simulink library "MuteRamperBtc"  (R2022b)
settings: Solver=VariableStepAuto  StartTime=0.0  StopTime=10.0  RelTol=1e-3
undefined symbols (not defined in the file or in its folder): InnerLinkConfig
libraries: AudioStats x1, FeaturePath x1, HandyTextFile x1, dspindex x1
settings Model: Creator=kl13806  LastModifiedBy=db1045444
settings SolverCC: AlgebraicLoopSolver=TrustRegion
settings DebuggingCC: UnconnectedInputMsg=warning  UnconnectedOutputMsg=warning  UnconnectedLineMsg=warning  SFMachineParentedDataDiag=warning
settings ModelReferenceCC: EnableRefExpFcnMdlSchedulingChecks=on
settings RTWCC: DLArmComputeVersion=19.05

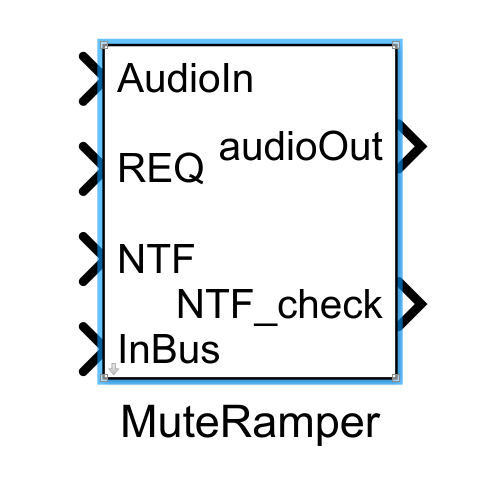
[thumbnail: Simulink's stored preview of the top-level diagram]
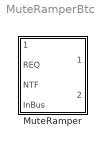
== system MuteRamperBtc ==
  MuteRamper : Subsystem  mask(Blocklib MuteRamper){Config=InnerLinkConfig, FeatureName=Mute}
      mask prompts: Config "MuteRamperConfig"; FeatureName "Feature path name:"
      mask help: This component is to be used in conjunction with the MuteControl block, which provides runtime control and tuning capabilities via an RTC and the tune variable muteControlRampTime. Multiple instances of this block may be placed within an audio application, and a single MuteControl block has the ability to control all of these rampers simultaneously.
      mask init:
      | blkh=gcbh;
      | Config=BTConfig.Assert(blkh,Config);
      | Config.Validate();
      | 
      | % Set boundary conditions
      | rampRateBounds = [5,50000];
      | rampTimeBounds = [1,3000];
      | 
      | % Setup Dsms
      | theDsms = {'currentGain','targetLinearGain','nFrames'};
      | CscUtil.SetupDsmsForStaticInit(blkh,theDsms);
      mask TypeOptions FeatureName: FeaturePath/FeatureName

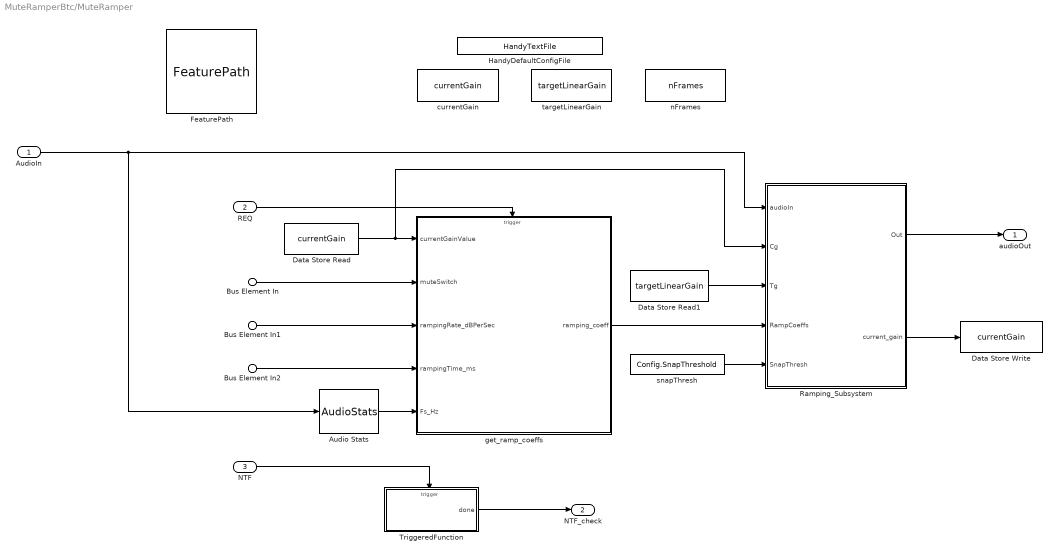
== system MuteRamperBtc/MuteRamper ==
  AudioIn : Inport
  REQ : Inport  Port=2
  NTF : Inport  Port=3
  Bus Element In : Inport  Port=4  PortName=InBus  Element=REQ_mute_switch
  Bus Element In1 : Inport  Port=4  PortName=InBus  Element=rampRate
  Bus Element In2 : Inport  Port=4  PortName=InBus  Element=rampTime
  Audio Stats : AudioStats/AudioStats  DoSampleRate=on  TypeSampleRate=Inherit: auto  DoCallRate=off  TypeCallRate=Inherit: auto  DoFrameSize=off  TypeFrameSize=Inherit: auto  DoChannelCount=off  TypeChannelCount=Inherit: auto  DoTaskRateFactor=off  TypeTaskRateFactor=Inherit: auto  MacroNameRoot=AUDIO  MacroNameRootEval='AUDIO'  IsMacroNameEval=off  MacroSampleRate=off  MacroCallRate=off  MacroFrameSize=off  MacroChannelCount=off  MacroTaskRateFactor=off  MacroTaskId=off  ValidateSampleRate=off  ValueSampleRate=[]  ValidateCallRate=off  ValueCallRate=[]  ValidateFrameSize=off  ValueFrameSize=[]  ValidateChannelCount=off  ValueChannelCount=[]  ValidateTaskRateFactor=off  ValueTaskRateFactor=[]
      settings: SourceProductName=Bose Talaria
  Data Store Read : DataStoreRead  DataStoreName=currentGain  IndexOptions=Index vector (dialog)  Indices=1  OutputSizes=1
  Data Store Read1 : DataStoreRead  DataStoreName=targetLinearGain  IndexOptions=Index vector (dialog)  Indices=1  OutputSizes=1
  Data Store Write : DataStoreWrite  DataStoreName=currentGain  IndexOptions=Index vector (dialog)  Indices=1  OutputSizes=1
  FeaturePath : FeaturePath/FeaturePath  FeatureName=Mute  IsGroup=off  GroupNumber=-1  IsModule=off  TriggerInit=[640 -31 755 76]
      settings: SourceProductName=Bose Talaria
  HandyDefaultConfigFile : HandyTextFile/HandyTextFile  TemplateSource=Config  FileSuffix=Init  OpenDialogOnLoad=off  UseThisBlockName=off  AddGrandParentNamePrefix=off  TheDefaultText=|  ShowInLibBrowser=on
      | % $(FILENAME) Setup model parameters for each "Init" callback (e.g. update diagram)
      | sample_rate_in_hertz = 44100;
      | frame_size = 32;
      | sysin_channel_count = 2;
      settings: SourceProductName=Bose Talaria
  Ramping_Subsystem : Subsystem  TreatAsAtomicUnit=on
  TriggeredFunction : MATLAB Function  TreatAsAtomicUnit=on
  currentGain : DataStoreMemory  DataStoreName=currentGain  InitialValue=Config.DlgInitialGainLinear  ShowAdditionalParam=off  OutDataTypeStr=single
  get_ramp_coeffs : MATLAB Function  TreatAsAtomicUnit=on  mask{silentGainLinear=Config.SilentGainLinear, frameSize=Config.SamplesPerFrame}
  nFrames : DataStoreMemory  DataStoreName=nFrames  ShowAdditionalParam=off  OutDataTypeStr=single
  snapThresh : Constant  Value=Config.SnapThreshold  VectorParams1D=off  OutDataTypeStr=single
  targetLinearGain : DataStoreMemory  DataStoreName=targetLinearGain  InitialValue=Config.DlgInitialGainLinear  ShowAdditionalParam=off  OutDataTypeStr=single
  audioOut : Outport  VectorParamsAs1DForOutWhenUnconnected=off
  NTF_check : Outport  Port=2
  wires:
  REQ/1 -> get_ramp_coeffs/Trigger
  snapThresh/1 -> Ramping_Subsystem/5(SnapThresh)
  Audio Stats/1 -> get_ramp_coeffs/5(Fs_Hz)
  NTF/1 -> TriggeredFunction/Trigger
  TriggeredFunction/1(done) -> NTF_check/1
  Bus Element In/1 -> get_ramp_coeffs/2(muteSwitch)
  Ramping_Subsystem/2(current_gain) -> Data Store Write/1
  Bus Element In2/1 -> get_ramp_coeffs/4(rampingTime_ms)
  Data Store Read1/1 -> Ramping_Subsystem/3(Tg)
  get_ramp_coeffs/1(ramping_coeff) -> Ramping_Subsystem/4(RampCoeffs)
  Ramping_Subsystem/1(Out) -> audioOut/1
  AudioIn/1 -> Audio Stats/1, Ramping_Subsystem/1(audioIn)
  Bus Element In1/1 -> get_ramp_coeffs/3(rampingRate_dBPerSec)
  Data Store Read/1 -> Ramping_Subsystem/2(Cg), get_ramp_coeffs/1(currentGainValue)

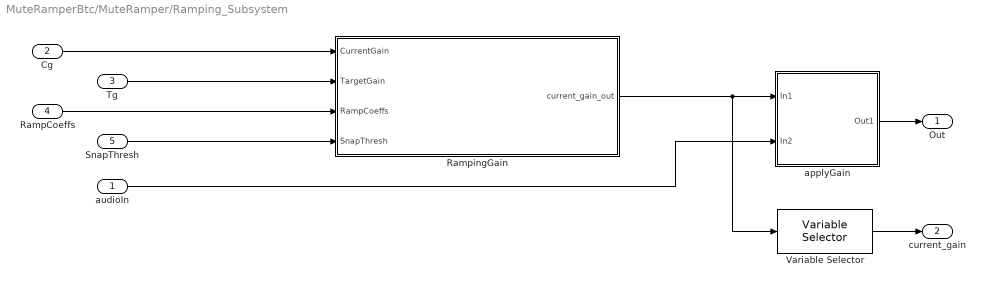
== system MuteRamperBtc/MuteRamper/Ramping_Subsystem ==
  audioIn : Inport
  Cg : Inport  Port=2
  Tg : Inport  Port=3
  RampCoeffs : Inport  Port=4
  SnapThresh : Inport  Port=5
  RampingGain : Subsystem
  Variable Selector : dspindex/Variable Selector  NumInputs=1  rowsOrCols=Rows  IdxMode=Fixed  Elements=Config.SamplesPerFrame  ZerOneIdxMode=One-based  errmode=Clip Index  FillMode=on  FillValues=0
  applyGain : Subsystem
  Out : Outport  VectorParamsAs1DForOutWhenUnconnected=off
  current_gain : Outport  Port=2  VectorParamsAs1DForOutWhenUnconnected=off
  wires:
  RampingGain/1(current_gain_out) -> applyGain/1(In1), Variable Selector/1
  audioIn/1 -> applyGain/2(In2)
  applyGain/1(Out1) -> Out/1
  Variable Selector/1 -> current_gain/1
  Cg/1 -> RampingGain/1(CurrentGain)
  SnapThresh/1 -> RampingGain/4(SnapThresh)
  Tg/1 -> RampingGain/2(TargetGain)
  RampCoeffs/1 -> RampingGain/3(RampCoeffs)

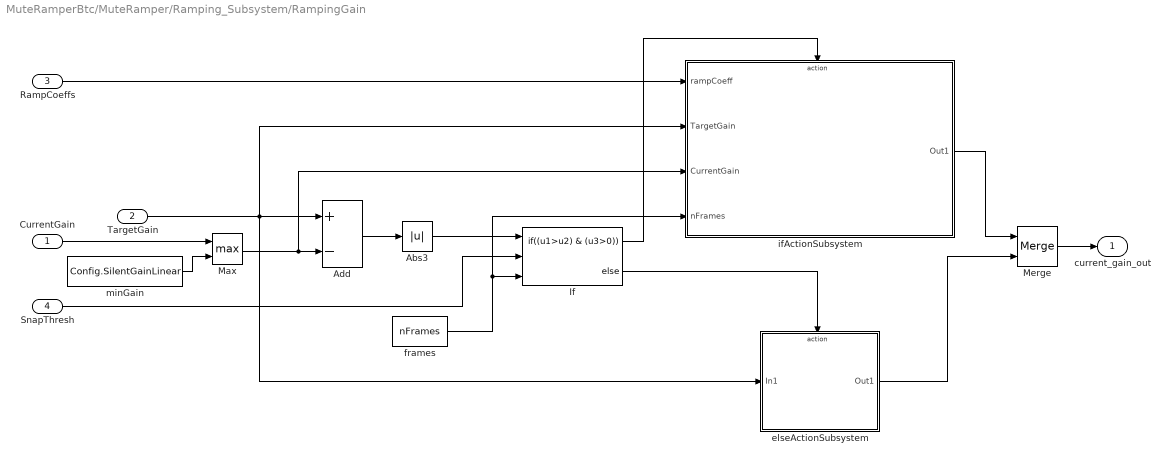
== system MuteRamperBtc/MuteRamper/Ramping_Subsystem/RampingGain ==
  CurrentGain : Inport
  TargetGain : Inport  Port=2
  RampCoeffs : Inport  Port=3
  SnapThresh : Inport  Port=4
  Abs3 : Abs  SaturateOnIntegerOverflow=off
  Add : Sum  Inputs=+-
  If : If  NumInputs=3  IfExpression=(u1>u2) & (u3>0)
  Max : MinMax  Function=max  Inputs=2
  Merge : Merge
  elseActionSubsystem : Subsystem
  frames : DataStoreRead  DataStoreName=nFrames  IndexOptions=Index vector (dialog)  Indices=1  OutputSizes=1
  ifActionSubsystem : Subsystem
  minGain : Constant  Value=Config.SilentGainLinear  OutDataTypeStr=single
  current_gain_out : Outport  VectorParamsAs1DForOutWhenUnconnected=off
  wires:
  Max/1 -> ifActionSubsystem/3(CurrentGain), Add/2
  Merge/1 -> current_gain_out/1
  Add/1 -> Abs3/1
  TargetGain/1 -> ifActionSubsystem/2(TargetGain), Add/1, elseActionSubsystem/1(In1)
  SnapThresh/1 -> If/2
  Abs3/1 -> If/1
  minGain/1 -> Max/2
  CurrentGain/1 -> Max/1
  If/1 -> ifActionSubsystem/Action
  If/2 -> elseActionSubsystem/Action
  RampCoeffs/1 -> ifActionSubsystem/1(rampCoeff)
  ifActionSubsystem/1(Out1) -> Merge/1
  elseActionSubsystem/1(Out1) -> Merge/2
  frames/1 -> ifActionSubsystem/4(nFrames), If/3

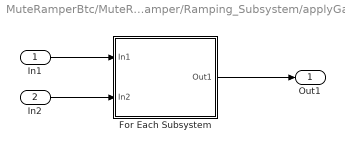
== system MuteRamperBtc/MuteRamper/Ramping_Subsystem/applyGain ==
  In1 : Inport
  In2 : Inport  Port=2
  For Each Subsystem : Subsystem  TreatAsAtomicUnit=on
  Out1 : Outport  VectorParamsAs1DForOutWhenUnconnected=off
  wires:
  In2/1 -> For Each Subsystem/2(In2)
  For Each Subsystem/1(Out1) -> Out1/1
  In1/1 -> For Each Subsystem/1(In1)

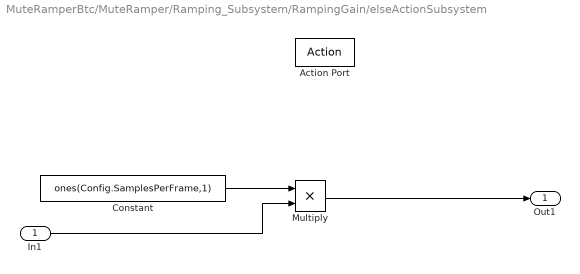
== system MuteRamperBtc/MuteRamper/Ramping_Subsystem/RampingGain/elseActionSubsystem ==
  In1 : Inport
  Action Port : ActionPort
  Constant : Constant  Value=ones(Config.SamplesPerFrame,1)  VectorParams1D=off  OutDataTypeStr=single
  Multiply : Product
  Out1 : Outport  VectorParamsAs1DForOutWhenUnconnected=off
  wires:
  Multiply/1 -> Out1/1
  In1/1 -> Multiply/2
  Constant/1 -> Multiply/1

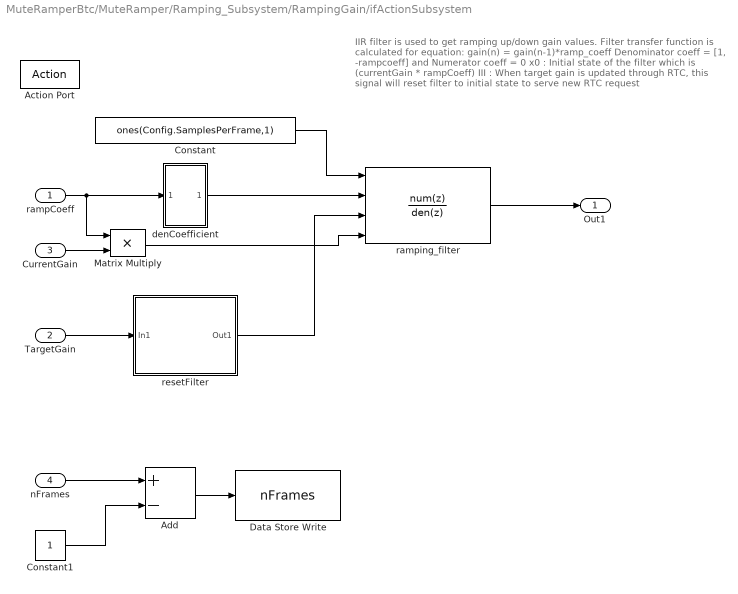
== system MuteRamperBtc/MuteRamper/Ramping_Subsystem/RampingGain/ifActionSubsystem ==
  note: IIR filter is used to get ramping up/down gain values. Filter transfer function
      |  is calculated for equation:
      | 	gain(n) = gain(n-1)*ramp_coeff
      |
      | Denominator coeff  = [1, -rampcoeff]  and Numerator coeff = 0
      | x0 : Initial state of the filter which is (currentGain * rampCoeff)
      | III : When target gain is updated through RTC, this signal will reset filter to
      | 	initial state to serve new RTC request
  rampCoeff : Inport
  TargetGain : Inport  Port=2
  CurrentGain : Inport  Port=3
  nFrames : Inport  Port=4
  Action Port : ActionPort
  Add : Sum  Inputs=+-
  Constant : Constant  Value=ones(Config.SamplesPerFrame,1)  VectorParams1D=off  OutDataTypeStr=single
  Constant1 : Constant  OutDataTypeStr=single
  Data Store Write : DataStoreWrite  DataStoreName=nFrames  IndexOptions=Index vector (dialog)  Indices=1  OutputSizes=1
  Matrix Multiply : Product
  denCoefficient : Subsystem
  ramping_filter : DiscreteFilter  Numerator=0  DenominatorSource=Input port  Denominator=[1 -1.0003]  InitialStatesSource=Input port  InitialStates=1.0003  InputProcessing=Columns as channels (frame based)  ExternalReset=Level hold  FilterStructure=Direct form II transposed  a0EqualsOne=on
      settings: InputPortMap=u0,p3,r7,p5
  resetFilter : Subsystem
  Out1 : Outport
  wires:
  TargetGain/1 -> resetFilter/1(In1)
  denCoefficient/1(Out1) -> ramping_filter/2
  resetFilter/1(Out1) -> ramping_filter/3
  rampCoeff/1 -> denCoefficient/1(In1), Matrix Multiply/1
  Constant/1 -> ramping_filter/1
  ramping_filter/1 -> Out1/1
  CurrentGain/1 -> Matrix Multiply/2
  Matrix Multiply/1 -> ramping_filter/4
  Add/1 -> Data Store Write/1
  Constant1/1 -> Add/2
  nFrames/1 -> Add/1

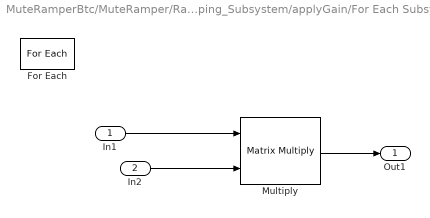
== system MuteRamperBtc/MuteRamper/Ramping_Subsystem/applyGain/For Each Subsystem ==
  In1 : Inport  Partition=on  PartitionDimension=1  PartitionWidth=1  PartitionOffset=0
  In2 : Inport  Port=2  Partition=on  PartitionDimension=1  PartitionWidth=1  PartitionOffset=0
  For Each : ForEach  DisableCoverage=on
  Multiply : Product  Multiplication=Matrix(*)
  Out1 : Outport  ConcatenationDimension=1
  wires:
  In1/1 -> Multiply/1
  In2/1 -> Multiply/2
  Multiply/1 -> Out1/1

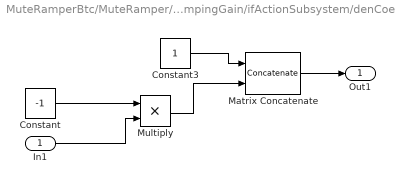
== system MuteRamperBtc/MuteRamper/Ramping_Subsystem/RampingGain/ifActionSubsystem/denCoefficient ==
  In1 : Inport
  Constant : Constant  Value=-1  OutDataTypeStr=single
  Constant3 : Constant  OutDataTypeStr=single
  Matrix Concatenate : Concatenate  Mode=Multidimensional array  ConcatenateDimension=2
  Multiply : Product
  Out1 : Outport  VectorParamsAs1DForOutWhenUnconnected=off
  wires:
  Constant3/1 -> Matrix Concatenate/1
  Matrix Concatenate/1 -> Out1/1
  Constant/1 -> Multiply/1
  Multiply/1 -> Matrix Concatenate/2
  In1/1 -> Multiply/2

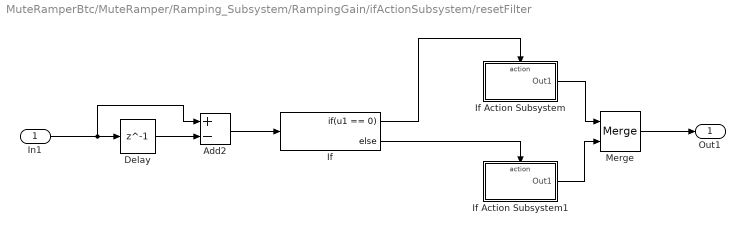
== system MuteRamperBtc/MuteRamper/Ramping_Subsystem/RampingGain/ifActionSubsystem/resetFilter ==
  In1 : Inport
  Add2 : Sum  Inputs=+-
  Delay : Delay  DelayLength=1
  If : If  IfExpression=u1 == 0
  If Action Subsystem : Subsystem  TreatAsAtomicUnit=on
  If Action Subsystem1 : Subsystem  TreatAsAtomicUnit=on
  Merge : Merge
  Out1 : Outport  VectorParamsAs1DForOutWhenUnconnected=off
  wires:
  Add2/1 -> If/1
  Delay/1 -> Add2/2
  In1/1 -> Add2/1, Delay/1
  If/1 -> If Action Subsystem/Action
  If/2 -> If Action Subsystem1/Action
  If Action Subsystem/1(Out1) -> Merge/1
  If Action Subsystem1/1(Out1) -> Merge/2
  Merge/1 -> Out1/1

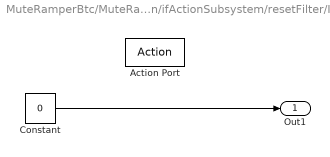
== system MuteRamperBtc/MuteRamper/Ramping_Subsystem/RampingGain/ifActionSubsystem/resetFilter/If Action Subsystem ==
  Action Port : ActionPort
  Constant : Constant  Value=0  OutDataTypeStr=boolean
  Out1 : Outport  VectorParamsAs1DForOutWhenUnconnected=off
  wires:
  Constant/1 -> Out1/1

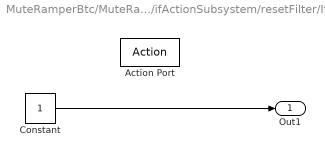
== system MuteRamperBtc/MuteRamper/Ramping_Subsystem/RampingGain/ifActionSubsystem/resetFilter/If Action Subsystem1 ==
  Action Port : ActionPort
  Constant : Constant  OutDataTypeStr=boolean
  Out1 : Outport  VectorParamsAs1DForOutWhenUnconnected=off
  wires:
  Constant/1 -> Out1/1

== matlab function MuteRamperBtc/MuteRamper/get_ramp_coeffs ==
  data: currentGainValue input; muteSwitch input; ramping_coeff output; rampingRate_dBPerSec input; rampingTime_ms input; Fs_Hz input; silentGainLinear parameter; targetLinearGain data_store_memory; nFrames data_store_memory; frameSize parameter
  events: trigger input FUNCTION_CALL_EVENT
function ramping_coeff = fcn(currentGainValue, muteSwitch, rampingRate_dBPerSec,rampingTime_ms, Fs_Hz, silentGainLinear, frameSize)

global targetLinearGain
global nFrames
targetLinearGain = single(1.0);

if muteSwitch
    targetLinearGain = single(max(0, silentGainLinear));
end

% % Nudge the gain values a bit if they are sitting at zero.
% % If current gain is zero, replace with a value very close to zero. What we
% % really want is a value which is on the edge of perception - not too small
% % or large. If the value is too small, we'll waste some of our ramp time
% % in perceived silence. If the value is too large, the audio will lurch
% % into perceptability at the start of the ramp.
% % So, 'max(currentGainValue, silentGainLinear)' & 'max(TargetGain, silentGainLinear)' are
% % used in equations

% In order to have the desired ramp time, the slope must vary dependent
% on the gain difference between target and current value.
% Equivalent ramp rate is therefore calculated as follows:

if (rampingRate_dBPerSec)
    currentGain_db = 20*log10(max(currentGainValue, silentGainLinear));
    targetGain_db = 20*log10( targetLinearGain);
    diff = abs(currentGain_db - targetGain_db);
    rampingTime_ms = diff / single(rampingRate_dBPerSec) * 1000;
end

quantum_ms = 1000 * frameSize / Fs_Hz;
numFrames = rampingTime_ms / quantum_ms;
% Do a ceil rather than a round to insure that we create enough
% frames. i.e. a fraction of a frame is promoted to an addition frame
nFrames = max (1, ceil(numFrames));
quantized_rampTime_ms = nFrames * quantum_ms;
   
% In order to have the desired ramp time, the slope must vary dependent
% on the gain differencebetween target and current value.
% Ramper's coefficient is therefore calculated as follows:
%
%   TargetGain = CurrentGain *( RampCoef ^ (Fs*RampTime_ms/1000) )
%
% therefore...
%
%                     log(TargetGain/CurrentGain)
%   log(RampCoef) = ------------------------------
%                        Fs*(RampTime_ms/1000)
%
ramping_coeff= exp(log( targetLinearGain /max(currentGainValue, silentGainLinear) ) / (Fs_Hz * quantized_rampTime_ms / 1000));

== matlab function MuteRamperBtc/MuteRamper/TriggeredFunction ==
  data: done output; targetLinearGain data_store_memory; currentGain data_store_memory
  events: trigger input FUNCTION_CALL_EVENT
function done = NotificationCheck()
% Function to check whether the ramp has completed. 
% If so, send out TRUE

global targetLinearGain;
global currentGain;

% Assume the work is complete until proven otherwise
done = true;
if (targetLinearGain ~= currentGain)
   done = false; % just proved otherwise
end
